simulink model "f01_CommRx1"  (R2024a)
settings: Solver=FixedStepDiscrete  StartTime=0.0  StopTime=1  FixedStep=mSim.dTime  MaxStep=Define.sModelSampleTime  RelTol=7.1420e-05
undefined symbols (not defined in the file): CRX1
settings Model: Creator=user  LastModifiedBy=admin
settings SolverCC: MaxConsecutiveZCs=10000  ZeroCrossAlgorithm=Adaptive  AlgebraicLoopSolver=TrustRegion
settings DataIOCC: SaveOutput=off  DSMLogging=off  InspectSignalLogs=on  SaveTime=off  SignalLoggingName=logsout_Validator
settings OptimizationCC: BlockReduction=off  DefaultParameterBehavior=Inlined  UseDivisionForNetSlopeComputation=UseDivisionForReciprocalsOfIntegersOnly  GainParamInheritBuiltInType=on  UseFloatMulNetSlope=on  DefaultUnderspecifiedDataType=single  InlineInvariantSignals=on  BitwiseOrLogicalOp=Logical operator  PassReuseOutputArgsAs=Individual arguments  EfficientFloat2IntCast=on  LifeSpan=Inf  OptimizeBlockOrder=speed  DifferentSizesBufferReuse=on  EfficientTunableParamExpr=on
settings DebuggingCC: SignalInfNanChecking=error  SignalRangeChecking=error  ReadBeforeWriteMsg=EnableAllAsError  WriteAfterWriteMsg=EnableAllAsError  WriteAfterReadMsg=EnableAllAsError  AlgebraicLoopMsg=error  ArtificialAlgebraicLoopMsg=error  SaveWithDisabledLinksMsg=error  SaveWithParameterizedLinksMsg=error  BlockPriorityViolationMsg=error  SolverPrmCheckMsg=error  InheritedTsInSrcMsg=error  SingleTaskRateTransMsg=error  TasksWithSamePriorityMsg=error  SigSpecEnsureSampleTimeMsg=error  CheckMatrixSingularityMsg=error  IntegerOverflowMsg=error  ParameterUnderflowMsg=error  ParameterPrecisionLossMsg=error  ParameterTunabilityLossMsg=error  UnderSpecifiedDataTypeMsg=error  UnnecessaryDatatypeConvMsg=warning  VectorMatrixConversionMsg=error  SignalLabelMismatchMsg=error  UnconnectedInputMsg=error  UnconnectedOutputMsg=error  UnconnectedLineMsg=error  SFcnCompatibilityMsg=error  UniqueDataStoreMsg=error  BusObjectLabelMismatch=error  RootOutportRequireBusObject=error  AssertControl=DisableAll  ModelReferenceIOMismatchMessage=error  UnknownTsInhSupMsg=error  ModelReferenceDataLoggingMessage=error  ModelReferenceSymbolNameMessage=none  StateNameClashWarn=warning  StrictBusMsg=ErrorOnBusTreatedAsVector  NonBusSignalsTreatedAsBus=error  SFInvalidInputDataAccessInChartInitDiag=error  SFTransitionOutsideNaturalParentDiag=error  SFUnreachableExecutionPathDiag=error  SFUndirectedBroadcastEventsDiag=error  SFTransitionActionBeforeConditionDiag=error  SFTemporalDelaySmallerThanSampleTimeDiag=error  SFSelfTransitionDiag=error  SFExecutionAtInitializationDiag=error  IntegerSaturationMsg=error  UnitsInconsistencyMsg=none  VariantConditionMismatch=error
settings HardwareCC: ProdBitPerChar=16  ProdBitPerInt=16  ProdBitPerPointer=32  ProdBitPerSizeT=32  ProdBitPerPtrDiffT=32  ProdLargestAtomicInteger=Integer  ProdLargestAtomicFloat=None  ProdWordSize=16  ProdHWDeviceType=Texas Instruments->C2000
settings ModelReferenceCC: EnableRefExpFcnMdlSchedulingChecks=on  ModelReferenceNumInstancesAllowed=Single
settings SFSimCC: SimUseLocalCustomCode=off  CompileTimeRecursionLimit=0  EnableRuntimeRecursion=off  MATLABDynamicMemAlloc=off  CustomCodeUndefinedFunction=UseInterfaceOnly
settings RTWCC: Description=Embedded Coder  SystemTargetFile=ert.tlc  GenCodeOnly=on  TemplateMakefile=ert_default_tmf  GenerateReport=on  RTWUseLocalCustomCode=off  CustomHeaderCode="#include \"Define_Header.h\""  BuildConfiguration=Faster Runs  IncludeHyperlinkInReport=on  LaunchReport=on  GenerateTraceInfo=on  GenerateTraceReport=on  GenerateTraceReportSl=on  GenerateTraceReportSf=on  GenerateWebview=on  GenerateCodeMetricsReport=on  GenerateCodeReplacementReport=on  GPUComputeCapability=3.5  DLArmComputeVersion=19.05
settings CodeAppCC: ForceParamTrailComments=on  IgnoreCustomStorageClasses=off  MATLABFcnDesc=on  MangleLength=4  CustomSymbolStrGlobalVar=GvF01$N$M  CustomSymbolStrType=StrF01$N$M  CustomSymbolStrFcn=$N$M$F  CustomSymbolStrMacro=$N$M  DefineNamingRule=UpperCase  ParamNamingRule=UpperCase  SimulinkBlockComments=off  MATLABSourceComments=on  EnableCustomComments=on  ReqsInCode=on
settings ERTTargetCC: TargetLangStandard=C99 (ISO)  UtilityFuncGeneration=Shared location  MultiwordLength=2048  IncludeMdlTerminateFcn=off  CombineSignalStateStructs=on  SuppressErrorStatus=on  SupportAbsoluteTime=off  SupportNonFinite=off  ParenthesesLevel=Maximum  CastingMode=Standards  GenerateSharedConstants=off  InlinedParameterPlacement=NonHierarchical  ERTSrcFileBannerTemplate=t_code_template.cgt  ERTHdrFileBannerTemplate=t_code_template.cgt  ERTDataSrcFileTemplate=t_code_template.cgt  ERTDataHdrFileTemplate=t_code_template.cgt  ERTCustomFileTemplate=example_file_process.tlc  ERTFilePackagingFormat=CompactWithDataFile  PreserveExpressionOrder=on  SuppressUnreachableDefaultCases=off  EnableSignedLeftShifts=off  EnableSignedRightShifts=off  IndentStyle=Allman  IndentSize=4
settings ConfigComp: CovSaveName=coveragedata  CovMetricSettings=we  CovEnableCumulative=off  CovSaveCumulativeToWorkspaceVar=on  CovSaveSingleToWorkspaceVar=on  CovOutputDir=sldv_output/$ModelName$\sldv_covoutput  PSVerificationMode=BugFinder  PSModelRefIgnoreList=[]  PSEnableModelRefIgnoreList=off  PSModelRefMinMaxVerif=CheckAndConstrain  PSAutoStubLUT=on  DVModelCoverageObjectives=MCDC  DVTestSuiteOptimization=CombinedObjectives (Nonlinear Extended)  DVRebuildModelRepresentation=Always
settings SimscapeCC: SimscapeNormalizeSystem=off

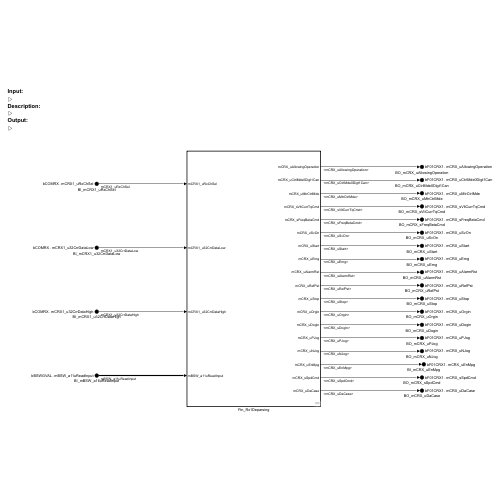
[thumbnail: Simulink's stored preview of the top-level diagram]
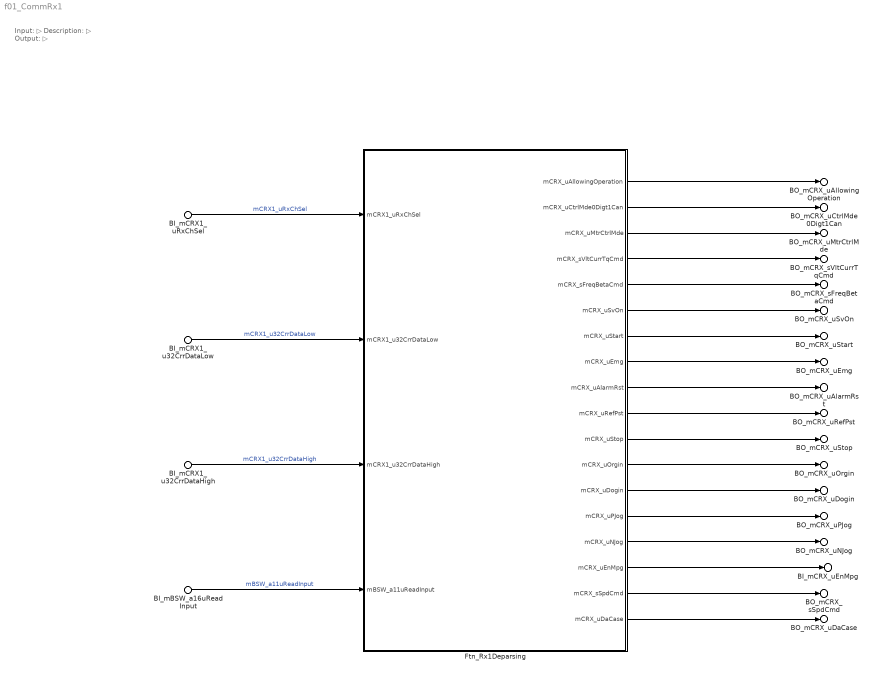
== system f01_CommRx1 ==
  note: Input:
      | ▷
      | Description:
      | ▷
      | Output:
      | ▷
  BI_mCRX1_uRxChSel : Inport  Description=■ 설명: 운전 모드 설정 (0: I/O, 1: 통신)  PortName=bCOMRX  Element=mCRX1_uRxChSel
  BI_mCRX1_u32CrrDataLow : Inport  Description=■ 설명: 통신 입력 Low 32bit  PortName=bCOMRX  Element=mCRX1_u32CrrDataLow
  BI_mCRX1_u32CrrDataHigh : Inport  Description=■ 설명: 통신 입력 High 32bit  PortName=bCOMRX  Element=mCRX1_u32CrrDataHigh
  BI_mBSW_a16uReadInput : Inport  Description=■ 설명: Digital Input Signal  Port=2  PortName=bBSWGVAL  Element=mBSW_a11uReadInput
  Ftn_Rx1Deparsing : Subsystem  TreatAsAtomicUnit=on
      settings: RTWSystemCode=Nonreusable function  RTWFcnNameOpts=Use subsystem name
  BO_mCRX_uAllowingOperation : Outport  Description=■ 설명: 통신 모드 구동 신호 (0: 미구동, 1: 구동)  PortName=bF01CRX1  Element=mCRX_uAllowingOperation
  BO_mCRX_uCtrlMde0Digt1Can : Outport  Description=■ 설명: Command Seletet (0: I/O, 1: CAN)  PortName=bF01CRX1  Element=mCRX_uCtrlMde0Digt1Can
  BO_mCRX_uMtrCtrlMde : Outport  Description=■ 설명: 모터 구동 모드 (1_VF/2_V/4_CURR/8_TQ/16_SPD/32_PST/64_VALIGN/128_ALIGN/256_IF)  PortName=bF01CRX1  Element=mCRX_uMtrCtrlMde
  BO_mCRX_sVltCurrTqCmd : Outport  Description=■ 설명: 통신 모드 구동 지령 (전압, 전류, 토크)  PortName=bF01CRX1  Element=mCRX_sVltCurrTqCmd
  BO_mCRX_sFreqBetaCmd : Outport  Description=■ 설명: 통신 모드 구동 지령 (주파수, 위상각)  PortName=bF01CRX1  Element=mCRX_sFreqBetaCmd
  BO_mCRX_uSvOn : Outport  Description=■ 설명: Digital Input Signal (서보 모터의 구동 신호, 0: 정지, 1: 구동)  PortName=bF01CRX1  Element=mCRX_uSvOn
  BO_mCRX_uStart : Outport  Description=■ 설명: Digital Input Signal (구동 시작 신호, 상승 엣지 후 100msec 이상 검출 시 활성화)  PortName=bF01CRX1  Element=mCRX_uStart
  BO_mCRX_uEmg : Outport  Description=■ 설명: Digital Input Signal (외부 비상 신호 입력, 0: 비상 신호 활성화, 1: 비상 신호 비활성화)  PortName=bF01CRX1  Element=mCRX_uEmg
  BO_mCRX_uAlarmRst : Outport  Description=■ 설명: Digital Input Signal (알람 및 경고 상태 해제 신호, 0: NA, 1: 해제)  PortName=bF01CRX1  Element=mCRX_uAlarmRst
  BO_mCRX_uRefPst : Outport  Description=■ 설명: Digital Input Signal (위치 데이터 입력 신호 6Bit Binary Code)  PortName=bF01CRX1  Element=mCRX_uRefPst
  BO_mCRX_uStop : Outport  Description=■ 설명: Digital Input Signal (동작 완료 신호)  PortName=bF01CRX1  Element=mCRX_uStop
  BO_mCRX_uOrgin : Outport  Description=■ 설명: Digital Input Signal (원점 설정 신호, 0: NA, 1: 원점 설정 활성화)  PortName=bF01CRX1  Element=mCRX_uOrgin
  BO_mCRX_uDogin : Outport  Description=■ 설명: Digital Input Signal (원점 설정 초기화 신호, 0: NA, 1: 원점 초기화 활성화)  PortName=bF01CRX1  Element=mCRX_uDogin
  BO_mCRX_uPJog : Outport  Description=■ 설명: Digital Input Signal (Manual CCW 구동 신호)  PortName=bF01CRX1  Element=mCRX_uPJog
  BO_mCRX_uNJog : Outport  Description=■ 설명: Digital Input Signal (Manual CW 구동 신호)  PortName=bF01CRX1  Element=mCRX_uNJog
  BI_mCRX_uEnMpg : Outport  Description=■ 설명: Digital Input Signal (미세 또는 단위 운전 설정, 0: 단위 운전, 1: 미세 운전)  PortName=bF01CRX1  Element=mCRX_uEnMpg
  BO_mCRX_sSpdCmd : Outport  Description=■ 설명: 통신 모드 속도 지령  PortName=bF01CRX1  Element=mCRX_sSpdCmd
  BO_mCRX_uDaCase : Outport  Description=■ 설명: DAC 출력 선택  PortName=bF01CRX1  Element=mCRX_uDaCase
  wires:
  BI_mCRX1_uRxChSel/1 -> Ftn_Rx1Deparsing/1(mCRX1_uRxChSel)  "mCRX1_uRxChSel"
  BI_mCRX1_u32CrrDataLow/1 -> Ftn_Rx1Deparsing/2(mCRX1_u32CrrDataLow)  "mCRX1_u32CrrDataLow"
  BI_mCRX1_u32CrrDataHigh/1 -> Ftn_Rx1Deparsing/3(mCRX1_u32CrrDataHigh)  "mCRX1_u32CrrDataHigh"
  BI_mBSW_a16uReadInput/1 -> Ftn_Rx1Deparsing/4(mBSW_a11uReadInput)  "mBSW_a11uReadInput"
  Ftn_Rx1Deparsing/11(mCRX_uStop) -> BO_mCRX_uStop/1
  Ftn_Rx1Deparsing/12(mCRX_uOrgin) -> BO_mCRX_uOrgin/1
  Ftn_Rx1Deparsing/13(mCRX_uDogin) -> BO_mCRX_uDogin/1
  Ftn_Rx1Deparsing/14(mCRX_uPJog) -> BO_mCRX_uPJog/1
  Ftn_Rx1Deparsing/15(mCRX_uNJog) -> BO_mCRX_uNJog/1
  Ftn_Rx1Deparsing/16(mCRX_uEnMpg) -> BI_mCRX_uEnMpg/1
  Ftn_Rx1Deparsing/17(mCRX_sSpdCmd) -> BO_mCRX_sSpdCmd/1
  Ftn_Rx1Deparsing/18(mCRX_uDaCase) -> BO_mCRX_uDaCase/1
  Ftn_Rx1Deparsing/4(mCRX_sVltCurrTqCmd) -> BO_mCRX_sVltCurrTqCmd/1
  Ftn_Rx1Deparsing/5(mCRX_sFreqBetaCmd) -> BO_mCRX_sFreqBetaCmd/1
  Ftn_Rx1Deparsing/6(mCRX_uSvOn) -> BO_mCRX_uSvOn/1
  Ftn_Rx1Deparsing/7(mCRX_uStart) -> BO_mCRX_uStart/1
  Ftn_Rx1Deparsing/8(mCRX_uEmg) -> BO_mCRX_uEmg/1
  Ftn_Rx1Deparsing/10(mCRX_uRefPst) -> BO_mCRX_uRefPst/1
  Ftn_Rx1Deparsing/1(mCRX_uAllowingOperation) -> BO_mCRX_uAllowingOperation/1
  Ftn_Rx1Deparsing/9(mCRX_uAlarmRst) -> BO_mCRX_uAlarmRst/1
  Ftn_Rx1Deparsing/3(mCRX_uMtrCtrlMde) -> BO_mCRX_uMtrCtrlMde/1
  Ftn_Rx1Deparsing/2(mCRX_uCtrlMde0Digt1Can) -> BO_mCRX_uCtrlMde0Digt1Can/1

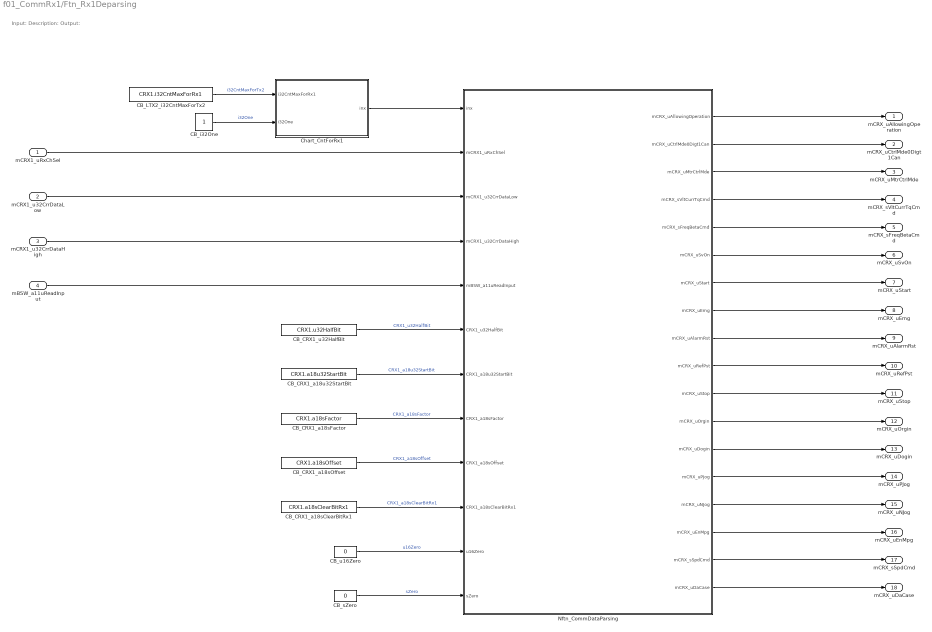
== system f01_CommRx1/Ftn_Rx1Deparsing ==
  note: Input:
      | Description:
      | Output:
  mCRX1_uRxChSel : Inport  OutMin=0  OutMax=1
  mCRX1_u32CrrDataLow : Inport  Port=2  OutMin=0  OutMax=4294967295
  mCRX1_u32CrrDataHigh : Inport  Port=3  OutMin=0  OutMax=4294967295
  mBSW_a11uReadInput : Inport  Port=4
  CB_CRX1_a18sClearBitRx1 : Constant  Value=CRX1.a18sClearBitRx1
  CB_CRX1_a18sFactor : Constant  Value=CRX1.a18sFactor
  CB_CRX1_a18sOffset : Constant  Value=CRX1.a18sOffset
  CB_CRX1_a18u32StartBit : Constant  Value=CRX1.a18u32StartBit
  CB_CRX1_u32HalfBit : Constant  Value=CRX1.u32HalfBit
  CB_LTX2_i32CntMaxForTx2 : Constant  Value=CRX1.i32CntMaxForRx1  OutDataTypeStr=int32
  CB_i32One : Constant  OutDataTypeStr=int32
  CB_sZero : Constant  Value=0  OutDataTypeStr=single
  CB_u16Zero : Constant  Value=0  OutDataTypeStr=uint16
  Chart_CntForRx1 : Stateflow chart  TreatAsAtomicUnit=on
  Nftn_CommDataParsing : Stateflow chart  TreatAsAtomicUnit=on  RTWFcnName=ftn_CommChartDataParsing
      settings: RTWSystemCode=Inline  RTWFcnNameOpts=Use subsystem name
  mCRX_uAllowingOperation : Outport
  mCRX_uCtrlMde0Digt1Can : Outport  Port=2
  mCRX_uMtrCtrlMde : Outport  Port=3
  mCRX_sVltCurrTqCmd : Outport  Port=4
  mCRX_sFreqBetaCmd : Outport  Port=5
  mCRX_uSvOn : Outport  Port=6
  mCRX_uStart : Outport  Port=7
  mCRX_uEmg : Outport  Port=8
  mCRX_uAlarmRst : Outport  Port=9
  mCRX_uRefPst : Outport  Port=10
  mCRX_uStop : Outport  Port=11
  mCRX_uOrgin : Outport  Port=12
  mCRX_uDogin : Outport  Port=13
  mCRX_uPJog : Outport  Port=14
  mCRX_uNJog : Outport  Port=15
  mCRX_uEnMpg : Outport  Port=16
  mCRX_sSpdCmd : Outport  Port=17
  mCRX_uDaCase : Outport  Port=18
  wires:
  CB_CRX1_a18sOffset/1 -> Nftn_CommDataParsing/9(CRX1_a18sOffset)  "CRX1_a18sOffset"
  mCRX1_uRxChSel/1 -> Nftn_CommDataParsing/2(mCRX1_uRxChSel)
  mCRX1_u32CrrDataLow/1 -> Nftn_CommDataParsing/3(mCRX1_u32CrrDataLow)
  CB_CRX1_a18sFactor/1 -> Nftn_CommDataParsing/8(CRX1_a18sFactor)  "CRX1_a18sFactor"
  CB_CRX1_a18u32StartBit/1 -> Nftn_CommDataParsing/7(CRX1_a18u32StartBit)  "CRX1_a18u32StartBit"
  CB_CRX1_a18sClearBitRx1/1 -> Nftn_CommDataParsing/10(CRX1_a18sClearBitRx1)  "CRX1_a18sClearBitRx1"
  CB_u16Zero/1 -> Nftn_CommDataParsing/11(u16Zero)  "u16Zero"
  CB_CRX1_u32HalfBit/1 -> Nftn_CommDataParsing/6(CRX1_u32HalfBit)  "CRX1_u32HalfBit"
  mCRX1_u32CrrDataHigh/1 -> Nftn_CommDataParsing/4(mCRX1_u32CrrDataHigh)
  CB_LTX2_i32CntMaxForTx2/1 -> Chart_CntForRx1/1(i32CntMaxForRx1)  "i32CntMaxForTx2"
  CB_i32One/1 -> Chart_CntForRx1/2(i32One)  "i32One"
  Chart_CntForRx1/1(inx) -> Nftn_CommDataParsing/1(inx)
  Nftn_CommDataParsing/9(mCRX_uAlarmRst) -> mCRX_uAlarmRst/1
  Nftn_CommDataParsing/1(mCRX_uAllowingOperation) -> mCRX_uAllowingOperation/1
  Nftn_CommDataParsing/3(mCRX_uMtrCtrlMde) -> mCRX_uMtrCtrlMde/1
  Nftn_CommDataParsing/4(mCRX_sVltCurrTqCmd) -> mCRX_sVltCurrTqCmd/1
  Nftn_CommDataParsing/5(mCRX_sFreqBetaCmd) -> mCRX_sFreqBetaCmd/1
  Nftn_CommDataParsing/6(mCRX_uSvOn) -> mCRX_uSvOn/1
  Nftn_CommDataParsing/7(mCRX_uStart) -> mCRX_uStart/1
  Nftn_CommDataParsing/8(mCRX_uEmg) -> mCRX_uEmg/1
  Nftn_CommDataParsing/10(mCRX_uRefPst) -> mCRX_uRefPst/1
  Nftn_CommDataParsing/11(mCRX_uStop) -> mCRX_uStop/1
  Nftn_CommDataParsing/12(mCRX_uOrgin) -> mCRX_uOrgin/1
  Nftn_CommDataParsing/13(mCRX_uDogin) -> mCRX_uDogin/1
  Nftn_CommDataParsing/14(mCRX_uPJog) -> mCRX_uPJog/1
  Nftn_CommDataParsing/15(mCRX_uNJog) -> mCRX_uNJog/1
  Nftn_CommDataParsing/16(mCRX_uEnMpg) -> mCRX_uEnMpg/1
  Nftn_CommDataParsing/17(mCRX_sSpdCmd) -> mCRX_sSpdCmd/1
  Nftn_CommDataParsing/18(mCRX_uDaCase) -> mCRX_uDaCase/1
  mBSW_a11uReadInput/1 -> Nftn_CommDataParsing/5(mBSW_a11uReadInput)
  CB_sZero/1 -> Nftn_CommDataParsing/12(sZero)  "sZero"
  Nftn_CommDataParsing/2(mCRX_uCtrlMde0Digt1Can) -> mCRX_uCtrlMde0Digt1Can/1

== stateflow chart f01_CommRx1/Ftn_Rx1Deparsing/Chart_CntForRx1 ==
  (default) -> (junction 2)
  (junction 2) -> (junction 3) [order 1] : [inx >= (i32CntMaxForRx1 - i32One)]
  (junction 2) -> (junction 13) [order 2] : {
      | inx = inx + i32One;
      | }
  (junction 3) -> (junction 4) : {
      | inx = Cnst_i32InitCntForRx1;
      | }
  (junction 4) -> (junction 13)
  (junction 13) -> (junction 34)
  data: inx output int32; Cnst_i32InitCntForRx1 constant int32 =0; i32CntMaxForRx1 input int32; i32One input

== stateflow chart f01_CommRx1/Ftn_Rx1Deparsing/Nftn_CommDataParsing ==
  note: Digital Input Signal
  note: Communication
  (default) -> (junction 163)
  (junction 163) -> (junction 242) [order 1] : [mCRX1_uRxChSel ~= u16Zero]
  (junction 163) -> (junction 295) [order 2] : {
      | mCRX_uAllowingOperation = u16Zero;
      | mCRX_uCtrlMde0Digt1Can = u16Zero;
      | mCRX_uMtrCtrlMde            = u16Zero;
      | mCRX_sVltCurrTqCmd       = sZero;
      | mCRX_sFreqBetaCmd        = sZero;
      | mCRX_uSvOn                     = mBSW_a11uReadInput[Cnst_i32_00];
      | mCRX_uStart                      = mBSW_a11uReadInput[Cnst_i32_01];
      | mCRX_uEmg                      = mBSW_a11uReadInput[Cnst_i32_02];
      | mCRX_uAlarmRst               = mBSW_a11uReadInput[Cnst_i32_03];
      | mCRX_uRefPst                   = mBSW_a11uReadInput[Cnst_i32_04];
      | mCRX_uStop                       = mBSW_a11uReadInput[Cnst_i32_05];
      | mCRX_uOrgin                      = mBSW_a11uReadInput[Cnst_i32_06];
      | mCRX_uDogin                     = mBSW_a11uReadInput[Cnst_i32_07];
      | mCRX_uPJog                      = mBSW_a11uReadInput[Cnst_i32_08];
      | mCRX_uNJog                      = mBSW_a11uReadInput[Cnst_i32_09];
      | mCRX_uEnMpg                   = mBSW_a11uReadInput[Cnst_i32_10];
      | mCRX_sSpdCmd                = sZero;
      | mCRX_uDaCase                 = u16Zero;
      | }
  (junction 242) -> (junction 380)
  (junction 380) -> (junction 382) [order 1] : [CRX1_a18u32StartBit[inx] >= CRX1_u32HalfBit]
  (junction 380) -> (junction 378) [order 2] : {
      | Local_u32CrrDataLow = uint32(mCRX1_u32CrrDataLow & CRX1_a18sClearBitRx1[inx]);
      | CRX1_u32Pars_Temp = uint32(Local_u32CrrDataLow>>CRX1_a18u32StartBit[inx]);
      | }
  (junction 382) -> (junction 381) : {
      | CRX1_u32High_StartBit = CRX1_a18u32StartBit[inx] - CRX1_u32HalfBit;
      | }
  (junction 381) -> (junction 379) : {
      | Local_u32CrrDataHigh = uint32(mCRX1_u32CrrDataHigh & CRX1_a18sClearBitRx1[inx]);
      | CRX1_u32Pars_Temp = uint32(Local_u32CrrDataHigh>>CRX1_u32High_StartBit);
      | }
  (junction 379) -> (junction 378)
  (junction 378) -> (junction 472) : {
      | sParsRlt1[inx] = (single(CRX1_u32Pars_Temp) * CRX1_a18sFactor[inx]) + CRX1_a18sOffset[inx];
      | }
  (junction 472) -> (junction 465) : {
      | mCRX_uDaCase = sParsRlt1[Cnst_i32_17];
      | mCRX_uCtrlMde0Digt1Can = sParsRlt1[Cnst_i32_01];
      | }
  (junction 465) -> (junction 467) [order 1] : [mCRX_uCtrlMde0Digt1Can == u16Zero]
  (junction 465) -> (junction 331) [order 2] : {
      | // CAN
      | mCRX_uAllowingOperation = sParsRlt1[Cnst_i32_00];
      | mCRX_uMtrCtrlMde            = sParsRlt1[Cnst_i32_02];
      | mCRX_sVltCurrTqCmd       = sParsRlt1[Cnst_i32_03];
      | mCRX_sFreqBetaCmd        = sParsRlt1[Cnst_i32_04];
      | mCRX_uSvOn                     = sParsRlt1[Cnst_i32_05];
      | mCRX_uStart                      = sParsRlt1[Cnst_i32_06];
      | mCRX_uEmg                      = sParsRlt1[Cnst_i32_07];
      | mCRX_uAlarmRst               = sParsRlt1[Cnst_i32_08];
      | mCRX_uRefPst                   = sParsRlt1[Cnst_i32_09];
      | mCRX_uStop                       = sParsRlt1[Cnst_i32_10];
      | mCRX_uOrgin                     = sParsRlt1[Cnst_i32_11];
      | mCRX_uDogin                     = sParsRlt1[Cnst_i32_12];
      | mCRX_uPJog                      = sParsRlt1[Cnst_i32_13];
      | mCRX_uNJog                      = sParsRlt1[Cnst_i32_14];
      | mCRX_uEnMpg                   = sParsRlt1[Cnst_i32_15];
      | mCRX_sSpdCmd                = sParsRlt1[Cnst_i32_16];
      | }
  (junction 467) -> (junction 468) : {
      | // I/O
      | mCRX_uAllowingOperation = u16Zero;
      | mCRX_uCtrlMde0Digt1Can = u16Zero;
      | mCRX_uMtrCtrlMde            = u16Zero;
      | mCRX_sVltCurrTqCmd       = sZero;
      | mCRX_sFreqBetaCmd        = sZero;
      | mCRX_uSvOn                     = mBSW_a11uReadInput[Cnst_i32_00];
      | mCRX_uStart                      = mBSW_a11uReadInput[Cnst_i32_01];
      | mCRX_uEmg                      = mBSW_a11uReadInput[Cnst_i32_02];
      | mCRX_uAlarmRst               = mBSW_a11uReadInput[Cnst_i32_03];
      | mCRX_uRefPst                   = mBSW_a11uReadInput[Cnst_i32_04];
      | mCRX_uStop                       = mBSW_a11uReadInput[Cnst_i32_05];
      | mCRX_uOrgin                      = mBSW_a11uReadInput[Cnst_i32_06];
      | mCRX_uDogin                     = mBSW_a11uReadInput[Cnst_i32_07];
      | mCRX_uPJog                      = mBSW_a11uReadInput[Cnst_i32_08];
      | mCRX_uNJog                      = mBSW_a11uReadInput[Cnst_i32_09];
      | mCRX_uEnMpg                   = mBSW_a11uReadInput[Cnst_i32_10];
      | mCRX_sSpdCmd                = sZero;
      | }
  (junction 468) -> (junction 331)
  (junction 331) -> (junction 295)
  (junction 295) -> (junction 334)
  data: inx input; mCRX1_uRxChSel input; mCRX1_u32CrrDataLow input; mCRX1_u32CrrDataHigh input; mBSW_a11uReadInput input uint16 size=11; CRX1_u32HalfBit input; CRX1_a18u32StartBit input size=18; CRX1_a18sFactor input size=18; CRX1_a18sOffset input size=18; CRX1_a18sClearBitRx1 input size=18; CRX1_u32Pars_Temp local uint32; CRX1_u32High_StartBit local uint32; sParsRlt1 local single size=[18 1]; u16Zero input; Local_u32CrrDataLow local uint32; Local_u32CrrDataHigh local uint32; mCRX_uAllowingOperation output uint16; mCRX_uCtrlMde0Digt1Can output uint16; mCRX_uMtrCtrlMde output uint16; mCRX_sVltCurrTqCmd output single; mCRX_sFreqBetaCmd output single; mCRX_uSvOn output uint16; mCRX_uStart output uint16; mCRX_uEmg output uint16; mCRX_uAlarmRst output uint16; mCRX_uRefPst output uint16; mCRX_uStop output uint16; mCRX_uOrgin output uint16; mCRX_uDogin output uint16; mCRX_uPJog output uint16; mCRX_uNJog output uint16; mCRX_uEnMpg output uint16; mCRX_sSpdCmd output single; mCRX_uDaCase output uint16; Cnst_i32_00 constant int32 =0; Cnst_i32_01 constant int32 =1; Cnst_i32_02 constant int32 =2; Cnst_i32_03 constant int32 =3; Cnst_i32_04 constant int32 =4; Cnst_i32_05 constant int32 =5; Cnst_i32_06 constant int32 =6; Cnst_i32_07 constant int32 =7; Cnst_i32_08 constant int32 =8; Cnst_i32_09 constant int32 =9; Cnst_i32_10 constant int32 =10; Cnst_i32_11 constant int32 =11; Cnst_i32_12 constant int32 =12; Cnst_i32_13 constant int32 =13; Cnst_i32_14 constant int32 =14; Cnst_i32_15 constant int32 =15; Cnst_i32_16 constant int32 =16; Cnst_i32_17 constant int32 =17; sZero input
